simulink model "Emf_Observer"  (R2023a)
settings: Solver=FixedStepAuto  StartTime=0.0  StopTime=10  FixedStep=0.0001  RelTol=1e-3  EnableMultiTasking=on
model workspace (MATLAB code in the model file + MAT data in the model file):
  cmdLim = Simulink.Parameter
  cmdLim.Value = 15
  cmdLim.Description = 'Limit for controlling the maximum surface command angle.'
  cmdLim.Min = 0
  cmdLim.Max = 90
  cmdLim.DocUnits = 'deg'
  dispGain = Simulink.Parameter
  dispGain.Value = 0.75
  dispGain.Description = 'Gain applied to the displacement error.'
  dispGain.Min = 0
  dispGain.Max = []
  dispGain.DocUnits = 'deg/sec/deg'
  dispLim = Simulink.Parameter
  dispLim.Value = 30
  dispLim.Description = 'Limit for controlling the maximum commanded angle.'
  dispLim.Min = 0
  dispLim.Max = 180
  dispLim.DocUnits = 'deg'
  intGain = Simulink.Parameter
  intGain.Value = 0.5
  intGain.Description = 'Gain applied to the integral error.'
  intGain.Min = 0
  intGain.Max = []
  intGain.DocUnits = 'deg/sec/deg/sec'
  intLim = Simulink.Parameter
  intLim.Value = 5
  intLim.Description = 'Limit for controlling the maximum commanded angle.'
  intLim.Min = 0
  intLim.Max = 90
  intLim.DocUnits = 'deg'
  rateGain = Simulink.Parameter
  rateGain.Value = 2
  rateGain.Description = 'Gain applied to the rate error.'
  rateGain.Min = 0
  rateGain.Max = []
  rateGain.DocUnits = 'deg/deg/sec'
  rateLim = Simulink.Parameter
  rateLim.Value = 6
  rateLim.Description = 'Limit for controlling the maximum commanded angle.'
  rateLim.Min = 0
  rateLim.Max = 180
  rateLim.DocUnits = 'deg/sec'
  hdgGain = Simulink.Parameter
  hdgGain.Value = 0.015
  VfSvc_EmfEstPiKi_Coef = Simulink.Parameter
  VfSvc_EmfEstPiKi_Coef.Value = 35.163
  VfSvc_EmfEstPiKi_Coef.DataType = 'single'
  VfSvc_EmfEstPiKi_Coef.Complexity = 'real'
  VfSvc_EmfEstPiKi_Coef.Dimensions = [1 1]
  VfSvc_EmfEstPiKp_Coef = Simulink.Parameter
  VfSvc_EmfEstPiKp_Coef.Value = 0.0194
  VfSvc_EmfEstPiKp_Coef.DataType = 'single'
  VfSvc_EmfEstPiKp_Coef.Complexity = 'real'
  VfSvc_EmfEstPiKp_Coef.Dimensions = [1 1]
  VfSvc_eSpeedEstPiKi_Coef = Simulink.Parameter
  VfSvc_eSpeedEstPiKi_Coef.Value = 35.163
  VfSvc_eSpeedEstPiKi_Coef.DataType = 'single'
  VfSvc_eSpeedEstPiKi_Coef.Complexity = 'real'
  VfSvc_eSpeedEstPiKi_Coef.Dimensions = [1 1]
  VfSvc_eSpeedEstPiKp_Coef = Simulink.Parameter
  VfSvc_eSpeedEstPiKp_Coef.Value = 0.0194
  VfSvc_eSpeedEstPiKp_Coef.DataType = 'single'
  VfSvc_eSpeedEstPiKp_Coef.Complexity = 'real'
  VfSvc_eSpeedEstPiKp_Coef.Dimensions = [1 1]
undefined symbols (not defined in the file): Flux, Ld, Lq, Rs
settings Model: RequirementInfo={} %GIDa_fe9045fd_0412_4b6e_8206_617cc20e6fde  Creator=洲  LastModifiedBy=洲
settings SolverCC: AlgebraicLoopSolver=TrustRegion  AutoInsertRateTranBlk=on
settings DataIOCC: SaveOutput=off  DSMLogging=off  SaveTime=off
settings OptimizationCC: DefaultParameterBehavior=Inlined  UseDivisionForNetSlopeComputation=on  GainParamInheritBuiltInType=on  UseFloatMulNetSlope=on  UseSpecifiedMinMax=on  InlineInvariantSignals=on  EnhancedBackFolding=on  PassReuseOutputArgsAs=Individual arguments  ZeroExternalMemoryAtStartup=off  ZeroInternalMemoryAtStartup=off  NoFixptDivByZeroProtection=on  EfficientFloat2IntCast=on  LifeSpan=1  OptimizeBlockOrder=speed  DifferentSizesBufferReuse=on  OptimizationCustomize=off  EfficientTunableParamExpr=on
settings DebuggingCC: MultiTaskRateTransMsg=warning  AllowSymbolicDim=off  SFUnexpectedBacktrackingDiag=warning  SFNoUnconditionalDefaultTransitionDiag=warning  SFExecutionAtInitializationDiag=none  ArithmeticOperatorsInVariantConditions=warning
settings HardwareCC: ProdLongLongMode=on
settings SFSimCC: MATLABDynamicMemAlloc=off
settings RTWCC: Description=Embedded Coder  SystemTargetFile=ert.tlc  GenCodeOnly=on  TemplateMakefile=ert_default_tmf  GenerateReport=on  BuildConfiguration=Faster Runs  IncludeHyperlinkInReport=on  LaunchReport=on  DataTypeReplacement=CDataTypesFixedWidth  GenerateTraceInfo=on  GenerateTraceReport=on  GenerateTraceReportSl=on  GenerateTraceReportSf=on  GenerateTraceReportEml=on  GenerateWebview=on  GenerateCodeMetricsReport=on  GenerateCodeReplacementReport=on
settings CodeAppCC: ForceParamTrailComments=on  IgnoreCustomStorageClasses=off  OperatorAnnotations=on  SimulinkDataObjDesc=on  SFDataObjDesc=on  CustomSymbolStrGlobalVar=rt$N$M  CustomSymbolStrType=$N$M  CustomSymbolStrFcn=$N$M$F  CustomSymbolStrMacro=$N$M  InsertBlockDesc=on  EnableCustomComments=on  ReqsInCode=on
settings ERTTargetCC: TargetLangStandard=C99 (ISO)  UtilityFuncGeneration=Shared location  MultiwordLength=2048  GenerateSampleERTMain=on  IncludeMdlTerminateFcn=off  CombineSignalStateStructs=on  SuppressErrorStatus=on  SupportAbsoluteTime=off  SupportNonFinite=off  SupportComplex=off  InlinedParameterPlacement=NonHierarchical  ERTCustomFileTemplate=example_file_process.tlc  ERTFilePackagingFormat=CompactWithDataFile
settings ConfigComp: CovScope=ReferencedModels  CovSaveName=covdata_rollAP  CovMetricSettings=dcmtrwe  CovHTMLOptions=-sRT=1 -aTS=1 -bRG=1 -bTC=1 -hTR=1 -nFC=0 -scm=1 -bcm=1 -xEv=0  CovSaveCumulativeToWorkspaceVar=on  CovSaveSingleToWorkspaceVar=on  CovCumulativeVarName=covCumulativeData_rollAP  CovReportOnPause=off  CovExternalEMLEnable=off  CovSFcnEnable=off

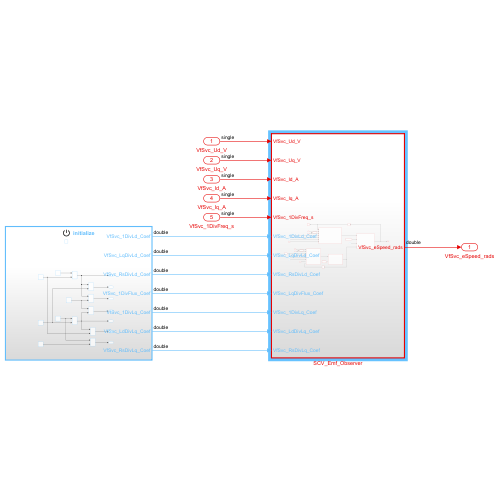
[thumbnail: Simulink's stored preview of the top-level diagram]
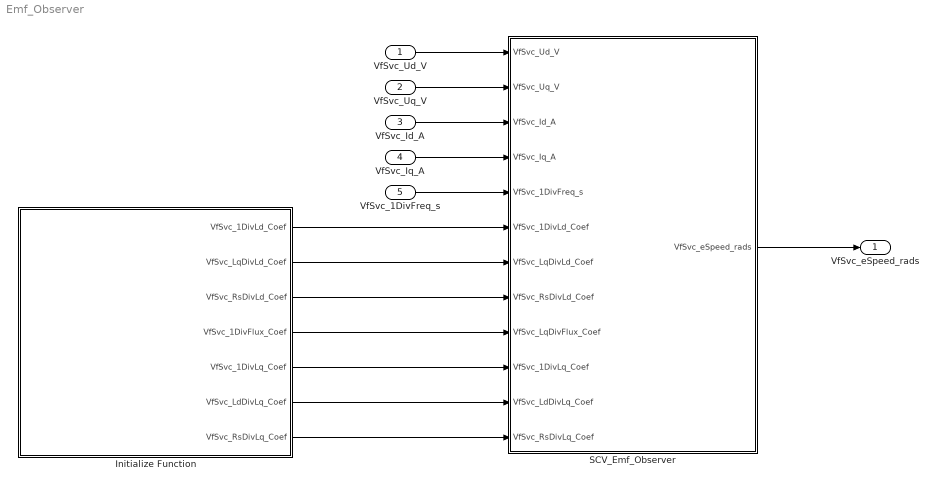
== system Emf_Observer ==
  VfSvc_Ud_V : Inport  OutDataTypeStr=single
  VfSvc_Uq_V : Inport  Port=2  OutDataTypeStr=single
  VfSvc_Id_A : Inport  Port=3  OutDataTypeStr=single
  VfSvc_Iq_A : Inport  Port=4  OutDataTypeStr=single
  VfSvc_1DivFreq_s : Inport  Port=5  OutDataTypeStr=single
  Initialize Function : Subsystem  TreatAsAtomicUnit=on
  SCV_Emf_Observer : Subsystem  TreatAsAtomicUnit=on
  VfSvc_eSpeed_rads : Outport
  wires:
  Initialize Function/1(VfSvc_1DivLd_Coef) -> SCV_Emf_Observer/6(VfSvc_1DivLd_Coef)
  Initialize Function/2(VfSvc_LqDivLd_Coef) -> SCV_Emf_Observer/7(VfSvc_LqDivLd_Coef)
  Initialize Function/3(VfSvc_RsDivLd_Coef) -> SCV_Emf_Observer/8(VfSvc_RsDivLd_Coef)
  Initialize Function/5(VfSvc_1DivLq_Coef) -> SCV_Emf_Observer/10(VfSvc_1DivLq_Coef)
  Initialize Function/6(VfSvc_LdDivLq_Coef) -> SCV_Emf_Observer/11(VfSvc_LdDivLq_Coef)
  Initialize Function/7(VfSvc_RsDivLq_Coef) -> SCV_Emf_Observer/12(VfSvc_RsDivLq_Coef)
  Initialize Function/4(VfSvc_1DivFlux_Coef) -> SCV_Emf_Observer/9(VfSvc_LqDivFlux_Coef)
  VfSvc_1DivFreq_s/1 -> SCV_Emf_Observer/5(VfSvc_1DivFreq_s)
  VfSvc_Ud_V/1 -> SCV_Emf_Observer/1(VfSvc_Ud_V)
  VfSvc_Uq_V/1 -> SCV_Emf_Observer/2(VfSvc_Uq_V)
  VfSvc_Id_A/1 -> SCV_Emf_Observer/3(VfSvc_Id_A)
  VfSvc_Iq_A/1 -> SCV_Emf_Observer/4(VfSvc_Iq_A)
  SCV_Emf_Observer/1(VfSvc_eSpeed_rads) -> VfSvc_eSpeed_rads/1

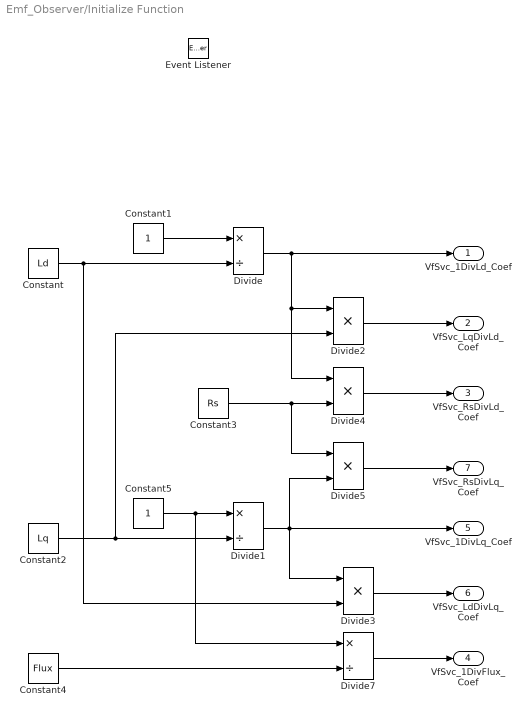
== system Emf_Observer/Initialize Function ==
  Constant : Constant  Value=Ld
  Constant1 : Constant
  Constant2 : Constant  Value=Lq
  Constant3 : Constant  Value=Rs
  Constant4 : Constant  Value=Flux
  Constant5 : Constant
  Divide : Product  Inputs=*/
  Divide1 : Product  Inputs=*/
  Divide{2..5} (4 alike) : Product  Inputs=**
  Divide7 : Product  Inputs=*/
  Event Listener : EventListener  DisableCoverage=on  EventName=reset
  VfSvc_1DivLd_Coef : Outport
  VfSvc_LqDivLd_Coef : Outport  Port=2
  VfSvc_RsDivLd_Coef : Outport  Port=3
  VfSvc_1DivFlux_Coef : Outport  Port=4
  VfSvc_1DivLq_Coef : Outport  Port=5
  VfSvc_LdDivLq_Coef : Outport  Port=6
  VfSvc_RsDivLq_Coef : Outport  Port=7
  wires:
  Constant1/1 -> Divide/1
  Divide/1 -> Divide4/1, Divide2/1, VfSvc_1DivLd_Coef/1
  Constant5/1 -> Divide7/1, Divide1/1
  Divide2/1 -> VfSvc_LqDivLd_Coef/1
  Divide1/1 -> Divide5/2, Divide3/1, VfSvc_1DivLq_Coef/1
  Divide3/1 -> VfSvc_LdDivLq_Coef/1
  Constant/1 -> Divide3/2, Divide/2
  Constant3/1 -> Divide5/1, Divide4/2
  Divide4/1 -> VfSvc_RsDivLd_Coef/1
  Divide5/1 -> VfSvc_RsDivLq_Coef/1
  Constant4/1 -> Divide7/2
  Constant2/1 -> Divide1/2, Divide2/2
  Divide7/1 -> VfSvc_1DivFlux_Coef/1

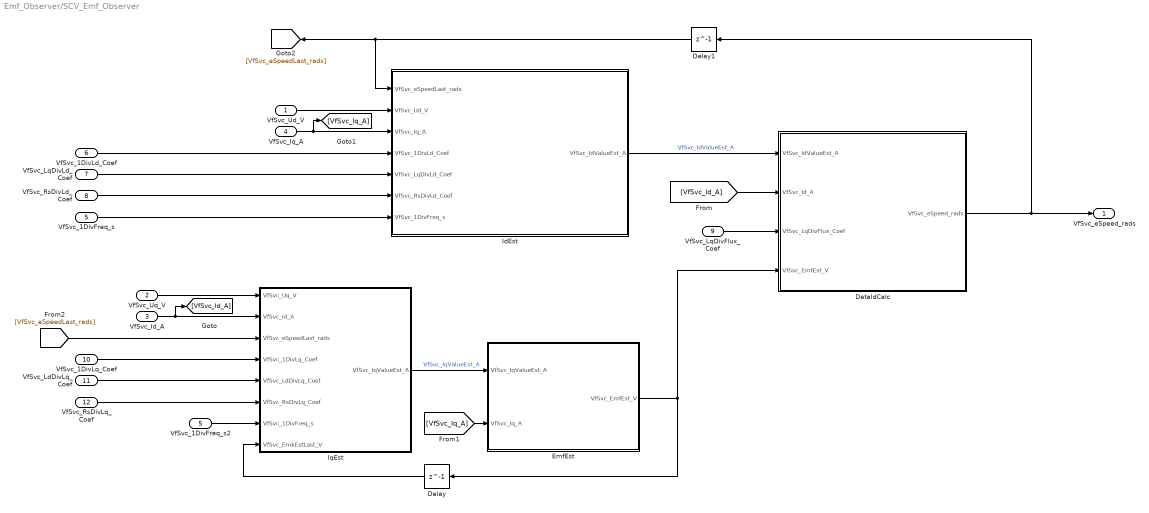
== system Emf_Observer/SCV_Emf_Observer ==
  VfSvc_Ud_V : Inport
  VfSvc_Uq_V : Inport  Port=2
  VfSvc_Id_A : Inport  Port=3
  VfSvc_Iq_A : Inport  Port=4
  VfSvc_1DivFreq_s : Inport  Port=5
  VfSvc_1DivLd_Coef : Inport  Port=6
  VfSvc_LqDivLd_Coef : Inport  Port=7
  VfSvc_RsDivLd_Coef : Inport  Port=8
  VfSvc_LqDivFlux_Coef : Inport  Port=9
  VfSvc_1DivLq_Coef : Inport  Port=10
  VfSvc_LdDivLq_Coef : Inport  Port=11
  VfSvc_RsDivLq_Coef : Inport  Port=12
  Delay : Delay  DelayLength=1
  Delay1 : Delay  DelayLength=1
  DetaIdCalc : Subsystem
  EmfEst : Subsystem
  IdEst : Subsystem  TreatAsAtomicUnit=on
      settings: RTWSystemCode=Nonreusable function  RTWFcnNameOpts=Use subsystem name
  IqEst : Subsystem  TreatAsAtomicUnit=on
      settings: RTWSystemCode=Nonreusable function  RTWFcnNameOpts=Use subsystem name
  VfSvc_1DivFreq_s2 : InportShadow  Port=5
  VfSvc_eSpeed_rads : Outport
  wires:
  VfSvc_Iq_A/1 -> [VfSvc_Iq_A], IdEst/3(VfSvc_Iq_A)
  DetaIdCalc/1(VfSvc_eSpeed_rads) -> Delay1/1, VfSvc_eSpeed_rads/1
  VfSvc_1DivLq_Coef/1 -> IqEst/4(VfSvc_1DivLq_Coef)
  [VfSvc_Iq_A] -> EmfEst/2(VfSvc_Iq_A)
  VfSvc_Uq_V/1 -> IqEst/1(VfSvc_Uq_V)
  Delay1/1 -> [VfSvc_eSpeedLast_rads], IdEst/1(VfSvc_eSpeedLast_rads)
  VfSvc_Id_A/1 -> IqEst/2(VfSvc_Id_A), [VfSvc_Id_A]
  EmfEst/1(VfSvc_EmfEst_V) -> DetaIdCalc/4(VfSvc_EmfEst_V), Delay/1
  Delay/1 -> IqEst/8(VfSvc_EmkEstLast_V)
  IdEst/1(VfSvc_IdValueEst_A) -> DetaIdCalc/1(VfSvc_IdValueEst_A)  "VfSvc_IdValueEst_A"
  VfSvc_LqDivFlux_Coef/1 -> DetaIdCalc/3(VfSvc_LqDivFlux_Coef)
  VfSvc_Ud_V/1 -> IdEst/2(VfSvc_Ud_V)
  [VfSvc_Id_A] -> DetaIdCalc/2(VfSvc_Id_A)
  VfSvc_RsDivLq_Coef/1 -> IqEst/6(VfSvc_RsDivLq_Coef)
  IqEst/1(VfSvc_IqValueEst_A) -> EmfEst/1(VfSvc_IqValueEst_A)  "VfSvc_IqValueEst_A"
  VfSvc_1DivFreq_s/1 -> IdEst/7(VfSvc_1DivFreq_s)
  VfSvc_LqDivLd_Coef/1 -> IdEst/5(VfSvc_LqDivLd_Coef)
  VfSvc_1DivLd_Coef/1 -> IdEst/4(VfSvc_1DivLd_Coef)
  VfSvc_LdDivLq_Coef/1 -> IqEst/5(VfSvc_LdDivLq_Coef)
  VfSvc_RsDivLd_Coef/1 -> IdEst/6(VfSvc_RsDivLd_Coef)
  VfSvc_1DivFreq_s2/1 -> IqEst/7(VfSvc_1DivFreq_s)
  [VfSvc_eSpeedLast_rads] -> IqEst/3(VfSvc_eSpeedLast_rads)

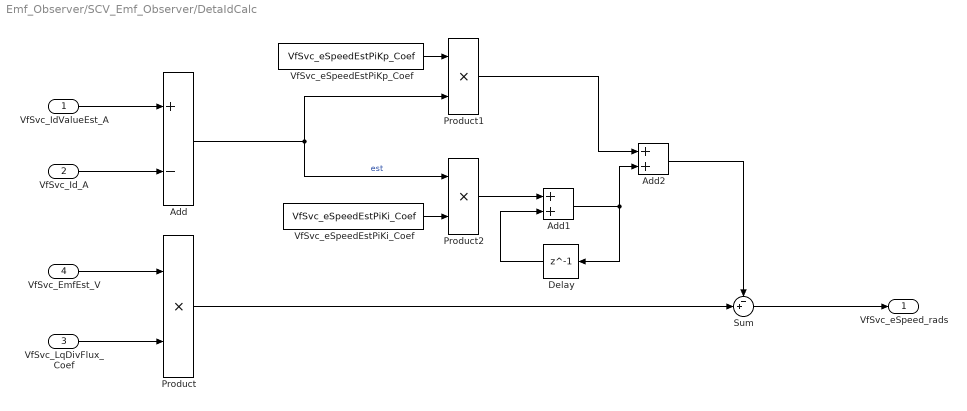
== system Emf_Observer/SCV_Emf_Observer/DetaIdCalc ==
  VfSvc_IdValueEst_A : Inport
  VfSvc_Id_A : Inport  Port=2
  VfSvc_LqDivFlux_Coef : Inport  Port=3
  VfSvc_EmfEst_V : Inport  Port=4
  Add : Sum  Inputs=+-
  Add1 : Sum
  Add2 : Sum
  Delay : Delay  DelayLength=1
  Product : Product
  Product1 : Product
  Product2 : Product
  Sum : Sum  Inputs=-+|
  VfSvc_eSpeedEstPiKi_Coef : Constant  Value=VfSvc_eSpeedEstPiKi_Coef
  VfSvc_eSpeedEstPiKp_Coef : Constant  Value=VfSvc_eSpeedEstPiKp_Coef
  VfSvc_eSpeed_rads : Outport
  wires:
  VfSvc_IdValueEst_A/1 -> Add/1
  VfSvc_Id_A/1 -> Add/2
  Product1/1 -> Add2/1
  Delay/1 -> Add1/2
  Add/1 -> Product1/2, Product2/1  "est"
  Add1/1 -> Delay/1, Add2/2
  Product2/1 -> Add1/1
  VfSvc_EmfEst_V/1 -> Product/1
  VfSvc_LqDivFlux_Coef/1 -> Product/2
  Product/1 -> Sum/2
  Add2/1 -> Sum/1
  Sum/1 -> VfSvc_eSpeed_rads/1
  VfSvc_eSpeedEstPiKp_Coef/1 -> Product1/1
  VfSvc_eSpeedEstPiKi_Coef/1 -> Product2/2

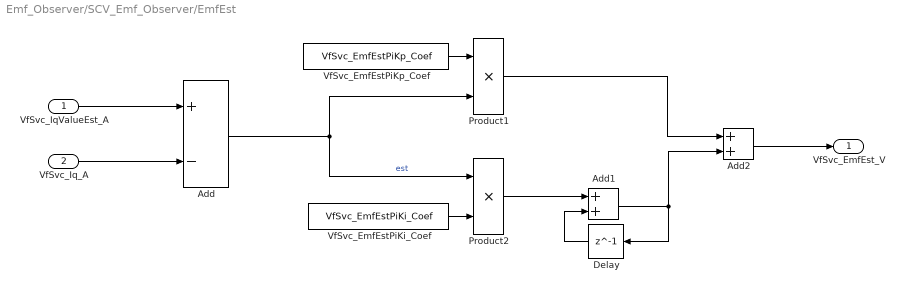
== system Emf_Observer/SCV_Emf_Observer/EmfEst ==
  VfSvc_IqValueEst_A : Inport
  VfSvc_Iq_A : Inport  Port=2
  Add : Sum  Inputs=+-
  Add1 : Sum
  Add2 : Sum
  Delay : Delay  DelayLength=1
  Product1 : Product
  Product2 : Product
  VfSvc_EmfEstPiKi_Coef : Constant  Value=VfSvc_EmfEstPiKi_Coef
  VfSvc_EmfEstPiKp_Coef : Constant  Value=VfSvc_EmfEstPiKp_Coef
  VfSvc_EmfEst_V : Outport
  wires:
  VfSvc_IqValueEst_A/1 -> Add/1
  VfSvc_Iq_A/1 -> Add/2
  Add2/1 -> VfSvc_EmfEst_V/1
  VfSvc_EmfEstPiKp_Coef/1 -> Product1/1
  Add/1 -> Product2/1, Product1/2  "est"
  VfSvc_EmfEstPiKi_Coef/1 -> Product2/2
  Product2/1 -> Add1/1
  Product1/1 -> Add2/1
  Add1/1 -> Delay/1, Add2/2
  Delay/1 -> Add1/2

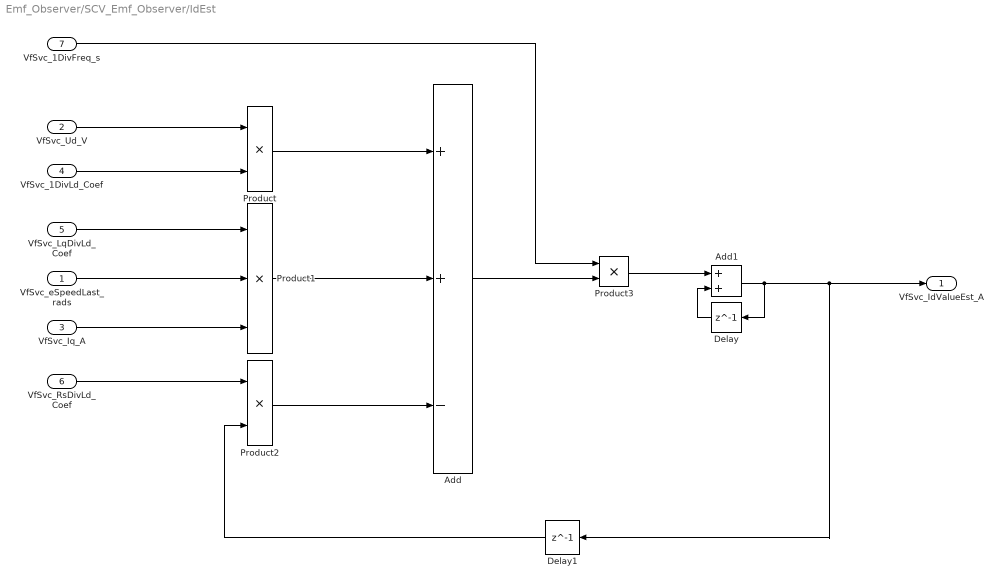
== system Emf_Observer/SCV_Emf_Observer/IdEst ==
  VfSvc_eSpeedLast_rads : Inport
  VfSvc_Ud_V : Inport  Port=2
  VfSvc_Iq_A : Inport  Port=3
  VfSvc_1DivLd_Coef : Inport  Port=4
  VfSvc_LqDivLd_Coef : Inport  Port=5
  VfSvc_RsDivLd_Coef : Inport  Port=6
  VfSvc_1DivFreq_s : Inport  Port=7
  Add : Sum  Inputs=++-
  Add1 : Sum
  Delay : Delay  DelayLength=1
  Delay1 : Delay  DelayLength=1
  Product : Product
  Product1 : Product  Inputs=3
  Product2 : Product
  Product3 : Product
  VfSvc_IdValueEst_A : Outport
  wires:
  VfSvc_Ud_V/1 -> Product/1
  VfSvc_1DivLd_Coef/1 -> Product/2
  VfSvc_LqDivLd_Coef/1 -> Product1/1
  VfSvc_eSpeedLast_rads/1 -> Product1/2
  VfSvc_Iq_A/1 -> Product1/3
  VfSvc_RsDivLd_Coef/1 -> Product2/1
  Product/1 -> Add/1
  Product1/1 -> Add/2
  Product2/1 -> Add/3
  Add/1 -> Product3/2
  VfSvc_1DivFreq_s/1 -> Product3/1
  Product3/1 -> Add1/1
  Add1/1 -> Delay1/1, VfSvc_IdValueEst_A/1, Delay/1
  Delay/1 -> Add1/2
  Delay1/1 -> Product2/2

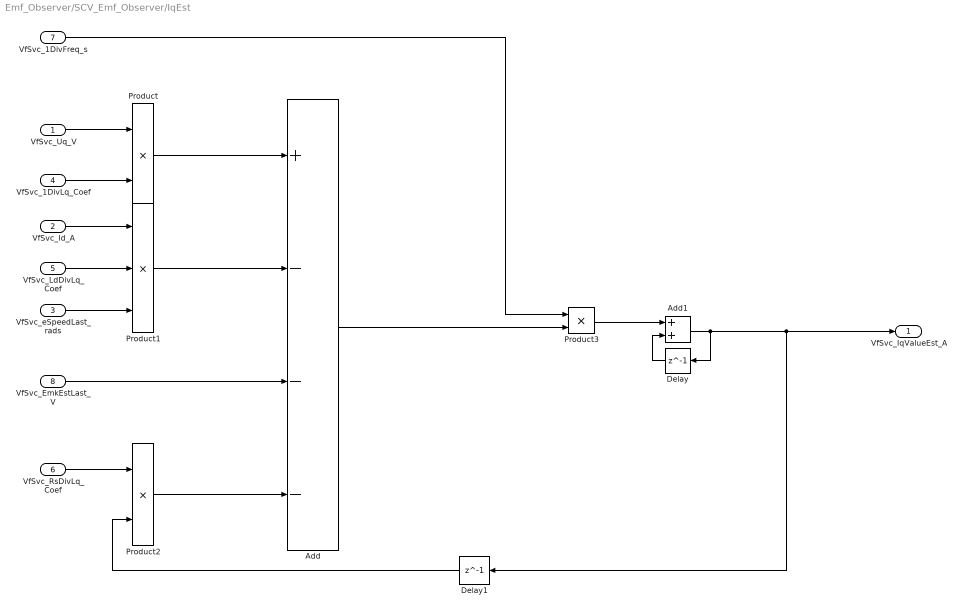
== system Emf_Observer/SCV_Emf_Observer/IqEst ==
  VfSvc_Uq_V : Inport
  VfSvc_Id_A : Inport  Port=2
  VfSvc_eSpeedLast_rads : Inport  Port=3
  VfSvc_1DivLq_Coef : Inport  Port=4
  VfSvc_LdDivLq_Coef : Inport  Port=5
  VfSvc_RsDivLq_Coef : Inport  Port=6
  VfSvc_1DivFreq_s : Inport  Port=7
  VfSvc_EmkEstLast_V : Inport  Port=8
  Add : Sum  Inputs=+---
  Add1 : Sum
  Delay : Delay  DelayLength=1
  Delay1 : Delay  DelayLength=1
  Product : Product
  Product1 : Product  Inputs=3
  Product2 : Product
  Product3 : Product
  VfSvc_IqValueEst_A : Outport
  wires:
  VfSvc_Uq_V/1 -> Product/1
  VfSvc_1DivLq_Coef/1 -> Product/2
  VfSvc_LdDivLq_Coef/1 -> Product1/2
  VfSvc_eSpeedLast_rads/1 -> Product1/3
  VfSvc_Id_A/1 -> Product1/1
  VfSvc_RsDivLq_Coef/1 -> Product2/1
  Product/1 -> Add/1
  Product1/1 -> Add/2
  VfSvc_EmkEstLast_V/1 -> Add/3
  Product2/1 -> Add/4
  Delay/1 -> Add1/2
  Add1/1 -> Delay1/1, VfSvc_IqValueEst_A/1, Delay/1
  VfSvc_1DivFreq_s/1 -> Product3/1
  Product3/1 -> Add1/1
  Add/1 -> Product3/2
  Delay1/1 -> Product2/2
